simulink library "TorqueCommand"  (R2025a)
settings: Solver=VariableStepAuto  StartTime=0.0  StopTime=10.0  RelTol=1e-3
values from neighbouring files (symbols this model uses):
  RegenEnable : value not decoded    [TorqueCommand.sldd]
  TCEnable : value not decoded    [TorqueCommand.sldd]
undefined symbols (not defined in the file or in its folder): DiscIntNeverNeededParam, dt, raptor_xcp_function, TorqueKiLowerSat, TorqueKiUpperSat
libraries: Raptor_lib x56, Utilities x14, simulink x7, $bdroot x5
(part 2 of 2)

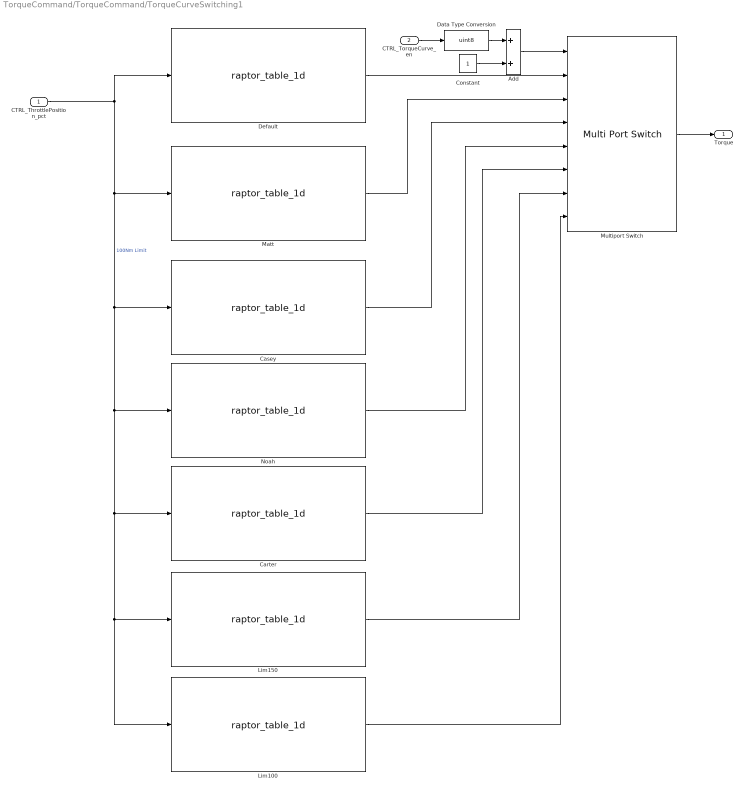
== system TorqueCommand/TorqueCommand/TorqueCurveSwitching1 ==
  CTRL_ThrottlePosition_pct : Inport
  CTRL_TorqueCurve_en : Inport  Port=2
  Add : Sum
  Carter : Raptor_lib/Table Lookup/raptor_table_1d  dataName='CTRL_ThrottleToTorqueCmdCarter_1D'  initValue=[0;1;3;6;11;18;25;34;45;57;70;85;101;118;137;158;179;202;227;230;230]  dataType=single  storage=Calibration  initValueX=[0;5;10;15;20;25;30;35;40;45;50;55;60;65;70;75;80;85;90;95;100]  dataTypeXY=single  storageXY=Calibration  calVisible=on  showTable=on  calGain=1.0  calOffset=0.0  calMax=Inf  calMin=-Inf  calFormat='-1'  calUnit='pct'  calHelp=''  showBreakpoint=on  dataNameX=[]  calGainX=1.0  calOffsetX=0.0  calMaxX=Inf  calMinX=-Inf  calFormatX='-1'  calUnitX='Nm'  calHelpX=''  calAccess=1  calFunction=raptor_xcp_function(gcb)  measureEnable=off  mName=['Data1D_Output']
      settings: SourceProductName=Raptor
  Casey : Raptor_lib/Table Lookup/raptor_table_1d  dataName='CTRL_ThrottleToTorqueCmdCasey_1D'  initValue=[0;3;6;9;12;15;25;35;45;55;65;75;85;95;105;115;135;155;175;195;200]  dataType=single  storage=Calibration  initValueX=[0;5;10;15;20;25;30;35;40;45;50;55;60;65;70;75;80;85;90;95;100]  dataTypeXY=single  storageXY=Calibration  calVisible=on  showTable=on  calGain=1.0  calOffset=0.0  calMax=Inf  calMin=-Inf  calFormat='-1'  calUnit='pct'  calHelp=''  showBreakpoint=on  dataNameX=[]  calGainX=1.0  calOffsetX=0.0  calMaxX=Inf  calMinX=-Inf  calFormatX='-1'  calUnitX='Nm'  calHelpX=''  calAccess=1  calFunction=raptor_xcp_function(gcb)  measureEnable=off  mName=['Data1D_Output']
      settings: SourceProductName=Raptor
  Constant : Constant
  Data Type Conversion : DataTypeConversion  OutDataTypeStr=uint8  SaturateOnIntegerOverflow=off  RndMeth=Floor
  Default : Raptor_lib/Table Lookup/raptor_table_1d  dataName='CTRL_ThrottleToTorqueCmdDef_1D'  initValue=[0;3;6;9;12;15;25;35;45;55;65;75;85;95;105;115;135;155;175;195;200]  dataType=single  storage=Calibration  initValueX=[0;5;10;15;20;25;30;35;40;45;50;55;60;65;70;75;80;85;90;95;100]  dataTypeXY=single  storageXY=Calibration  calVisible=on  showTable=on  calGain=1.0  calOffset=0.0  calMax=Inf  calMin=-Inf  calFormat='-1'  calUnit='pct'  calHelp=''  showBreakpoint=on  dataNameX=[]  calGainX=1.0  calOffsetX=0.0  calMaxX=Inf  calMinX=-Inf  calFormatX='-1'  calUnitX='Nm'  calHelpX=''  calAccess=1  calFunction=raptor_xcp_function(gcb)  measureEnable=off  mName=['Data1D_Output']
      settings: SourceProductName=Raptor
  Lim100 : Raptor_lib/Table Lookup/raptor_table_1d  dataName='CTRL_ThrottleToTorqueCmd100_1D'  initValue=[0;8;17;25;33;40;48;55;62;68;74;79;84;88;92;95;97;99;100;100;100]  dataType=single  storage=Calibration  initValueX=[0;5;10;15;20;25;30;35;40;45;50;55;60;65;70;75;80;85;90;95;100]  dataTypeXY=single  storageXY=Calibration  calVisible=on  showTable=on  calGain=1.0  calOffset=0.0  calMax=Inf  calMin=-Inf  calFormat='-1'  calUnit='pct'  calHelp=''  showBreakpoint=on  dataNameX=[]  calGainX=1.0  calOffsetX=0.0  calMaxX=Inf  calMinX=-Inf  calFormatX='-1'  calUnitX='Nm'  calHelpX=''  calAccess=1  calFunction=raptor_xcp_function(gcb)  measureEnable=off  mName=['Data1D_Output']
      settings: SourceProductName=Raptor
  Lim150 : Raptor_lib/Table Lookup/raptor_table_1d  dataName='CTRL_ThrottleToTorqueCmd150_1D'  initValue=[0;8;17;25;33;40;48;55;62;68;74;79;84;88;92;95;97;99;100;100;100]  dataType=single  storage=Calibration  initValueX=[0;5;10;15;20;25;30;35;40;45;50;55;60;65;70;75;80;85;90;95;100]  dataTypeXY=single  storageXY=Calibration  calVisible=on  showTable=on  calGain=1.0  calOffset=0.0  calMax=Inf  calMin=-Inf  calFormat='-1'  calUnit='pct'  calHelp=''  showBreakpoint=on  dataNameX=[]  calGainX=1.0  calOffsetX=0.0  calMaxX=Inf  calMinX=-Inf  calFormatX='-1'  calUnitX='Nm'  calHelpX=''  calAccess=1  calFunction=raptor_xcp_function(gcb)  measureEnable=off  mName=['Data1D_Output']
      settings: SourceProductName=Raptor
  Matt : Raptor_lib/Table Lookup/raptor_table_1d  dataName='CTRL_ThrottleToTorqueCmdMatt_1D'  initValue=[0;3;6;9;12;15;25;35;45;55;65;75;85;95;105;115;135;155;175;195;200]  dataType=single  storage=Calibration  initValueX=[0;5;10;15;20;25;30;35;40;45;50;55;60;65;70;75;80;85;90;95;100]  dataTypeXY=single  storageXY=Calibration  calVisible=on  showTable=on  calGain=1.0  calOffset=0.0  calMax=Inf  calMin=-Inf  calFormat='-1'  calUnit='pct'  calHelp=''  showBreakpoint=on  dataNameX=[]  calGainX=1.0  calOffsetX=0.0  calMaxX=Inf  calMinX=-Inf  calFormatX='-1'  calUnitX='Nm'  calHelpX=''  calAccess=1  calFunction=raptor_xcp_function(gcb)  measureEnable=off  mName=['Data1D_Output']
      settings: SourceProductName=Raptor
  Multiport Switch : MultiPortSwitch  Inputs=7  SaturateOnIntegerOverflow=off  InputSameDT=off
  Noah : Raptor_lib/Table Lookup/raptor_table_1d  dataName='CTRL_ThrottleToTorqueCmdNoah_1D'  initValue=[0;3;6;9;12;15;25;35;45;55;65;75;85;95;105;115;135;155;175;195;200]  dataType=single  storage=Calibration  initValueX=[0;5;10;15;20;25;30;35;40;45;50;55;60;65;70;75;80;85;90;95;100]  dataTypeXY=single  storageXY=Calibration  calVisible=on  showTable=on  calGain=1.0  calOffset=0.0  calMax=Inf  calMin=-Inf  calFormat='-1'  calUnit='pct'  calHelp=''  showBreakpoint=on  dataNameX=[]  calGainX=1.0  calOffsetX=0.0  calMaxX=Inf  calMinX=-Inf  calFormatX='-1'  calUnitX='Nm'  calHelpX=''  calAccess=1  calFunction=raptor_xcp_function(gcb)  measureEnable=off  mName=['Data1D_Output']
      settings: SourceProductName=Raptor
  Torque : Outport
  wires:
  Data Type Conversion/1 -> Add/1
  Constant/1 -> Add/2
  Add/1 -> Multiport Switch/1
  CTRL_TorqueCurve_en/1 -> Data Type Conversion/1
  Multiport Switch/1 -> Torque/1
  Lim100/1 -> Multiport Switch/8
  Lim150/1 -> Multiport Switch/7
  Carter/1 -> Multiport Switch/6
  Noah/1 -> Multiport Switch/5
  Casey/1 -> Multiport Switch/4
  Matt/1 -> Multiport Switch/3
  Default/1 -> Multiport Switch/2
  CTRL_ThrottlePosition_pct/1 -> Default/1, Matt/1, Casey/1, Noah/1, Carter/1, Lim100/1, Lim150/1  "100Nm Limit"

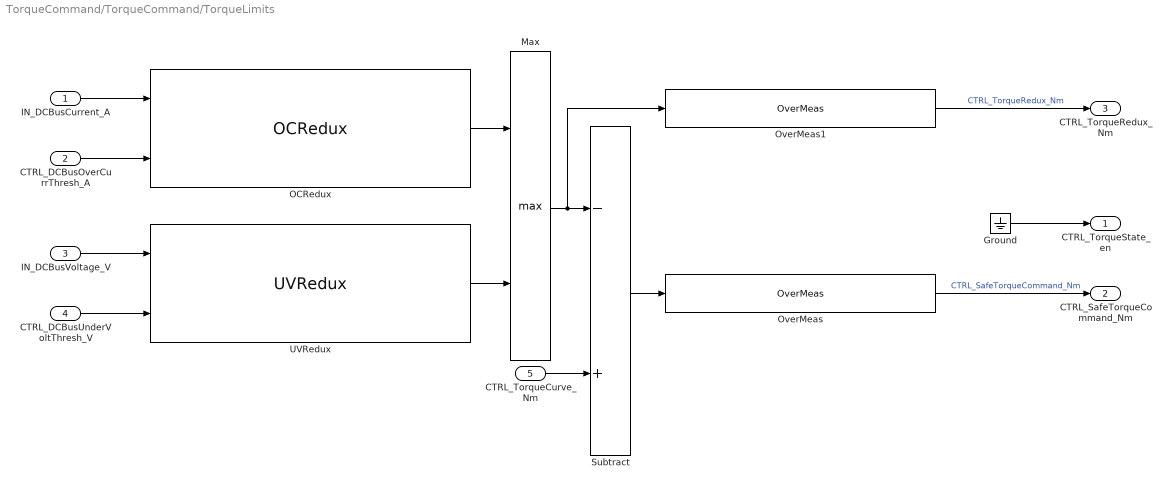
== system TorqueCommand/TorqueCommand/TorqueLimits ==
  IN_DCBusCurrent_A : Inport
  CTRL_DCBusOverCurrThresh_A : Inport  Port=2
  IN_DCBusVoltage_V : Inport  Port=3
  CTRL_DCBusUnderVoltThresh_V : Inport  Port=4
  CTRL_TorqueCurve_Nm : Inport  Port=5
  Ground : Ground
  Max : MinMax  Function=max  Inputs=2
  OCRedux : $bdroot/OCRedux  SystemSampleTime=-1  VariantActivationTime=update diagram  EmptyChoice=off  PassThrough=off  PassThroughVariantControl=(default)  EmptyChoiceVariantControl=(default)  AllowFlexibleInterface=on  Latency=0  AutoFrameSizeCalculation=off
  OverMeas : Utilities/OverMeas  sigName='CTRL_SafeTorqueCommand_Nm'  minimum=-inf  maximum=inf
  OverMeas1 : Utilities/OverMeas  sigName='CTRL_TorqueRedux_Nm'  minimum=-inf  maximum=inf
  Subtract : Sum  Inputs=-+
  UVRedux : $bdroot/UVRedux  SystemSampleTime=-1  VariantActivationTime=update diagram  EmptyChoice=off  PassThrough=off  PassThroughVariantControl=(default)  EmptyChoiceVariantControl=(default)  AllowFlexibleInterface=on  Latency=0  AutoFrameSizeCalculation=off
  CTRL_TorqueState_en : Outport
  CTRL_SafeTorqueCommand_Nm : Outport  Port=2
  CTRL_TorqueRedux_Nm : Outport  Port=3
  wires:
  OverMeas1/1 -> CTRL_TorqueRedux_Nm/1  "CTRL_TorqueRedux_Nm"
  Ground/1 -> CTRL_TorqueState_en/1
  CTRL_DCBusUnderVoltThresh_V/1 -> UVRedux/2
  IN_DCBusVoltage_V/1 -> UVRedux/1
  UVRedux/1 -> Max/2
  OverMeas/1 -> CTRL_SafeTorqueCommand_Nm/1  "CTRL_SafeTorqueCommand_Nm"
  Subtract/1 -> OverMeas/1
  CTRL_TorqueCurve_Nm/1 -> Subtract/2
  Max/1 -> Subtract/1, OverMeas1/1
  CTRL_DCBusOverCurrThresh_A/1 -> OCRedux/2
  IN_DCBusCurrent_A/1 -> OCRedux/1
  OCRedux/1 -> Max/1

== matlab function TorqueCommand/ShifterState/MATLAB Function ==
  data: IO_PwrUpSwitch_bool input; IO_PwrDownSwitch_bool input; stateNum output
function stateNum = fcn(IO_PwrUpSwitch_bool, IO_PwrDownSwitch_bool)
 
persistent state prevUp prevDown
 
if isempty(state)

    state = TorqueState.State5;

end

if isempty(prevUp)

    prevUp = false;

    prevDown = false;

end
 
upButton = logical(IO_PwrUpSwitch_bool);

downButton = logical(IO_PwrDownSwitch_bool);
 
upEdge = (upButton && ~prevUp);

downEdge = (downButton && ~prevDown);
 
if upEdge

    newValue = min(uint8(state) + 1, 5);

    state = TorqueState(newValue);

elseif downEdge

    newValue = max(uint8(state) - 1, 0);

    state = TorqueState(newValue);

end
 
stateNum = uint8(state);
 
prevUp = upButton;

prevDown = downButton;

== stateflow chart TorqueCommand/TorqueProfiles/Chart ==
  state VehicleStatic
    state Default
      entry:
      Profile = TorqueProfile.Player1;
      Curve = TorqueCurve.Default;
      TC = TCEnable.TCOff;
      Regen = RegenEnable.RegOff;
      Sensitivity = 5;
    state Testing2
      entry:
      Profile = TorqueProfile.Testing2;
      Curve = TorqueCurve.Lim100;
      TC = TCEnable.TCOn;
      Regen = RegenEnable.RegOn;
      Sensitivity = 5;
    state Driver1
      entry:
      Profile = TorqueProfile.Driver1;
      Curve = TorqueCurve.Matt;
      TC = TCEnable.TCOn;
      Regen = RegenEnable.RegOn;
      Sensitivity = 5;
    state Testing3
      entry:
      Profile = TorqueProfile.Testing3;
      Curve = TorqueCurve.Default;
      TC = TCEnable.TCOn;
      Regen = RegenEnable.RegOn;
      Sensitivity = 0;
    state Driver2
      entry:
      Profile = TorqueProfile.Driver2;
      Curve = TorqueCurve.Casey;
      TC = TCEnable.TCOn;
      Regen = RegenEnable.RegOn;
      Sensitivity = 5;
    state Testing4
      entry:
      Profile = TorqueProfile.Testing4;
      Curve = TorqueCurve.Default;
      TC = TCEnable.TCOn;
      Regen = RegenEnable.RegOn;
      Sensitivity = 1;
    state Driver3
      entry:
      Profile = TorqueProfile.Driver3;
      Curve = TorqueCurve.Noah;
      TC = TCEnable.TCOn;
      Regen = RegenEnable.RegOn;
      Sensitivity = 5;
    state Testing5
      entry:
      Profile = TorqueProfile.Testing5;
      Curve = TorqueCurve.Default;
      TC = TCEnable.TCOn;
      Regen = RegenEnable.RegOn;
      Sensitivity = 2;
    state Driver4
      entry:
      Profile = TorqueProfile.Driver4;
      Curve = TorqueCurve.Carter;
      TC = TCEnable.TCOn;
      Regen = RegenEnable.RegOn;
      Sensitivity = 5;
    state Testing6
      entry:
      Profile = TorqueProfile.Testing6;
      Curve = TorqueCurve.Default;
      TC = TCEnable.TCOn;
      Regen = RegenEnable.RegOn;
      Sensitivity = 3;
    state Testing1
      entry:
      Profile = TorqueProfile.Testing1;
      Curve = TorqueCurve.Lim150;
      TC = TCEnable.TCOn;
      Regen = RegenEnable.RegOn;
      Sensitivity = 5;
    (default) -> Default
    (junction 264) -> Default : [TCDial == 0]
    Testing2 -> (junction 276) : [TCDial ~= 6]
    (junction 47) -> (junction 264) [order 1]
    (junction 276) -> (junction 47)
    Default -> (junction 287) : [TCDial ~= 0]
    (junction 289) -> Testing2 : [TCDial == 6]
    (junction 287) -> (junction 47)
    (junction 47) -> (junction 289) [order 7]
    (junction 282) -> Driver1 : [TCDial == 1]
    Testing3 -> (junction 284) : [TCDial ~= 7]
    (junction 47) -> (junction 282) [order 2]
    (junction 284) -> (junction 47)
    Driver1 -> (junction 283) : [TCDial ~= 1]
    (junction 285) -> Testing3 : [TCDial == 7]
    (junction 283) -> (junction 47)
    (junction 47) -> (junction 285) [order 8]
    Testing4 -> (junction 269) : [TCDial ~= 8]
    (junction 273) -> Driver2 : [TCDial == 2]
    (junction 47) -> (junction 273) [order 3]
    (junction 269) -> (junction 47)
    (junction 274) -> (junction 47)
    (junction 47) -> (junction 267) [order 9]
    (junction 267) -> Testing4 : [TCDial == 8]
    (junction 47) -> (junction 271) [order 4]
    (junction 277) -> (junction 47)
    Driver2 -> (junction 274) : [TCDial ~= 2]
    (junction 272) -> (junction 47)
    (junction 47) -> (junction 278) [order 10]
    (junction 47) -> (junction 270) [order 5]
    (junction 280) -> (junction 47)
    (junction 268) -> (junction 47)
    (junction 47) -> (junction 279) [order 11]
    (junction 47) -> (junction 263) [order 6] : [TCDial == 5]
    (junction 281) -> (junction 47) : [TCDial ~= 5]
    (junction 271) -> Driver3 : [TCDial == 3]
    Testing5 -> (junction 277) : [TCDial ~= 9]
    Driver3 -> (junction 272) : [TCDial ~= 3]
    (junction 278) -> Testing5 : [TCDial == 9]
    (junction 270) -> Driver4 : [TCDial == 4]
    Testing6 -> (junction 280) : [TCDial ~= 10]
    Driver4 -> (junction 268) : [TCDial ~= 4]
    (junction 279) -> Testing6 : [TCDial == 10]
    (junction 263) -> Testing1
    Testing1 -> (junction 281)
  state ReadyToMove
    state NoTC
      entry:
      Sensitivity = 1;
    state Sens6
      entry:
      Sensitivity = 6;
    state Sens7
      entry:
      Sensitivity = 7;
    state Sens1
      entry:
      Sensitivity = 2;
    state Sens2
      entry:
      Sensitivity = 2;
    state Sens8
      entry:
      Sensitivity = 8;
    state Sens3
      entry:
      Sensitivity = 3;
    state Sens9
      entry:
      Sensitivity = 9;
    state Sens4
      entry:
      Sensitivity = 4;
    state Sens10
      entry:
      Sensitivity = 10;
    state Sens5
      entry:
      Sensitivity = 5;
    (default) -> NoTC
    (junction 395) -> NoTC : [TCDial == 0]
    Sens6 -> (junction 391) : [TCDial ~= 6]
    (junction 403) -> (junction 395) [order 1]
    (junction 391) -> (junction 403)
    NoTC -> (junction 396) : [TCDial ~= 0]
    (junction 397) -> Sens6 : [TCDial == 6]
    (junction 396) -> (junction 403)
    (junction 403) -> (junction 397) [order 7]
    (junction 390) -> Sens1 : [TCDial == 1]
    Sens7 -> (junction 392) : [TCDial ~= 7]
    (junction 403) -> (junction 390) [order 2]
    (junction 392) -> (junction 403)
    Sens1 -> (junction 394) : [TCDial ~= 1]
    (junction 393) -> Sens7 : [TCDial == 7]
    (junction 394) -> (junction 403)
    (junction 403) -> (junction 393) [order 8]
    Sens8 -> (junction 398) : [TCDial ~= 8]
    (junction 402) -> Sens2 : [TCDial == 2]
    (junction 403) -> (junction 402) [order 3]
    (junction 398) -> (junction 403)
    (junction 399) -> (junction 403)
    (junction 403) -> (junction 407) [order 9]
    (junction 407) -> Sens8 : [TCDial == 8]
    (junction 403) -> (junction 400) [order 4]
    (junction 401) -> (junction 403)
    Sens2 -> (junction 399) : [TCDial ~= 2]
    (junction 404) -> (junction 403)
    (junction 403) -> (junction 405) [order 10]
    (junction 403) -> (junction 406) [order 5]
    (junction 408) -> (junction 403)
    (junction 409) -> (junction 403)
    (junction 403) -> (junction 413) [order 11]
    (junction 403) -> (junction 410) [order 6]
    (junction 411) -> (junction 403)
    (junction 400) -> Sens3 : [TCDial == 3]
    Sens9 -> (junction 401) : [TCDial ~= 9]
    Sens3 -> (junction 404) : [TCDial ~= 3]
    (junction 405) -> Sens9 : [TCDial == 9]
    (junction 406) -> Sens4 : [TCDial == 4]
    Sens10 -> (junction 408) : [TCDial ~= 10]
    Sens4 -> (junction 409) : [TCDial ~= 4]
    (junction 413) -> Sens10 : [TCDial == 10]
    (junction 410) -> Sens5 : [TCDial == 5]
    Sens5 -> (junction 411) : [TCDial ~= 5]
  (default) -> VehicleStatic
  VehicleStatic -> ReadyToMove : [[State == VehicleState.ReadyToMove]]
  ReadyToMove -> VehicleStatic : [State ~= VehicleState.ReadyToMove]
  data: Profile output; Curve output; Sensitivity output; TCDial input; State input; Regen output; TC output

== stateflow chart TorqueCommand/BrakeRegen/Chart ==
  state RegenOff
    en:
    RegenMode = 0;
  state RegenOn
    state RegenMode1
      en:
      RegenMode = 1;
      RegenCoefficient = 1;
    state RegenMode2
      en:
      RegenMode = 2;
      RegenCoefficient = 1.5;
    state RegenMode4
      en:
      RegenMode = 4;
      RegenCoefficient = 2.5;
    state RegenMode3
      en:
      RegenMode = 3;
      RegenCoefficient = 2;
    state RegenMode5
      en:
      RegenMode = 5;
      RegenCoefficient = 3;
    state RegenMode6
      en:
      RegenMode = 6;
      RegenCoefficient = 3.5;
    state RegenMode7
      en:
      RegenMode = 7;
      RegenCoefficient = CTRL_RegenCoefficient_int;
    (default) -> RegenMode1
    RegenMode2 -> RegenMode1 [order 1] : [CTRL_DebPwrDown_int == 1]
    RegenMode1 -> RegenMode2 : [CTRL_DebPwrUp_int == 1]
    RegenMode3 -> RegenMode2 [order 1] : [CTRL_DebPwrDown_int == 1]
    RegenMode2 -> RegenMode3 [order 2] : [CTRL_DebPwrUp_int == 1]
    RegenMode3 -> RegenMode4 [order 2] : [CTRL_DebPwrUp_int == 1]
    RegenMode4 -> RegenMode3 [order 1] : [CTRL_DebPwrDown_int == 1]
    RegenMode5 -> RegenMode4 [order 1] : [CTRL_DebPwrDown_int == 1]
    RegenMode4 -> RegenMode5 [order 2] : [CTRL_DebPwrUp_int == 1]
    RegenMode5 -> RegenMode6 [order 2] : [CTRL_DebPwrUp_int == 1]
    RegenMode6 -> RegenMode5 [order 1] : [CTRL_DebPwrDown_int == 1]
    RegenMode7 -> RegenMode6 : [CTRL_DebPwrDown_int == 1]
    RegenMode6 -> RegenMode7 [order 2] : [CTRL_DebPwrUp_int == 1]
  (default) -> RegenOff
  RegenOn -> RegenOff : [Regen == RegenEnable.RegOff && ...
      |  IN_DCBusVolt_V > 370 && ...
      | CTRL_ThrottlePosition_pct > 5 && ...
      | IN_MotorSpeed_rpm < 700]
  RegenOff -> RegenOn : [Regen == RegenEnable.RegOn && ...
      | IN_DCBusVolt_V <= 370 && ...
      | CTRL_ThrottlePosition_pct <= 5 && ...
      | IN_MotorSpeed_rpm >= 700]
  data: Regen input; IN_DCBusVolt_V input; CTRL_ThrottlePosition_pct input; CTRL_DebPwrUp_int input; CTRL_DebPwrDown_int input; RegenMode output; RegenCoefficient output; CTRL_RegenCoefficient_int input; IN_MotorSpeed_rpm input

== stateflow chart TorqueCommand/TorqueCeiling ==
  state Default
    en:
    State = TorqueCeiling.NA;
    Torque = 230;
  state UnderVoltage
    en:
    State = TorqueCeiling.UnderVoltage;
    state UnderVoltInit
      en:
      Torque = 100;
    state UnderVolt3
      en:
      Torque = 50;
    state UnderVolt2
      en:
      Torque = 50;
    (default) -> UnderVoltInit
    UnderVoltInit -> UnderVolt3 : [DCBusVolts >= UnderVoltageThreshold]
    UnderVolt3 -> UnderVolt2 : [DCBusVolts >= UnderVoltageThreshold]
  state OverCurrent1
    en:
    State = TorqueCeiling.OverCurr;
    state OverCurrInit
      en:
      Torque = 100;
    state OverCurr2
      en:
      Torque = 70;
    state OverCurr3
      en:
      Torque = 50;
    (default) -> OverCurrInit
    OverCurrInit -> OverCurr2 : [DCBusCurrent >= OverCurrentThreshold]
    OverCurr2 -> OverCurr3 : [DCBusCurrent >= OverCurrentThreshold]
  (default) -> Default
  Default -> (junction 31) [order 2] : [DCBusVolts >= UnderVoltageThreshold]
  Default -> (junction 18) [order 1] : [DCBusCurrent >= OverCurrentThreshold]
  (junction 31) -> UnderVoltage
  (junction 18) -> OverCurrent1
  (junction 34) -> Default
  UnderVoltage -> (junction 34) : [ThrottlePosition <= 50]
  OverCurrent1 -> (junction 34) : [ThrottlePosition <= 50]
  data: DCBusVolts input; DCBusCurrent input; ThrottlePosition input; UnderVoltageThreshold input; OverCurrentThreshold input; State output; Torque output

== matlab function TorqueCommand/BrakeRegen/MATLAB Function ==
  data: IO_PwrUpSwitch_bool input; CTRL_DebPwrUp_int output; IO_PwrDownSwitch_bool input; dt input; CTRL_DebPwrDown_int output
function [CTRL_DebPwrUp_int, CTRL_DebPwrDown_int] = debouncePowerButtons(IO_PwrUpSwitch_bool, IO_PwrDownSwitch_bool, dt)
% Debounce two power buttons
%
% Inputs:
%   IO_PwrUpSwitch_bool   - raw Power Up button input
%   IO_PwrDownSwitch_bool - raw Power Down button input
%   dt                    - sample time in seconds
%
% Outputs:
%   CTRL_DebPwrUp_int     - debounced Power Up button
%   CTRL_DebPwrDown_int   - debounced Power Down button

    persistent upOut upLastRaw upCount
    persistent downOut downLastRaw downCount

    debounceTime = 0.03;   % 30 ms debounce
    nDebounce = max(1, ceil(debounceTime / dt));

    if isempty(upOut)
        upOut = logical(IO_PwrUpSwitch_bool);
        upLastRaw = logical(IO_PwrUpSwitch_bool);
        upCount = 0;

        downOut = logical(IO_PwrDownSwitch_bool);
        downLastRaw = logical(IO_PwrDownSwitch_bool);
        downCount = 0;
    end

    % -------- Power Up debounce --------
    rawUp = logical(IO_PwrUpSwitch_bool);

    if rawUp ~= upLastRaw
        upLastRaw = rawUp;
        upCount = 1;
    else
        upCount = upCount + 1;
    end

    if rawUp ~= upOut && upCount >= nDebounce
        upOut = rawUp;
    end

    % -------- Power Down debounce --------
    rawDown = logical(IO_PwrDownSwitch_bool);

    if rawDown ~= downLastRaw
        downLastRaw = rawDown;
        downCount = 1;
    else
        downCount = downCount + 1;
    end

    if rawDown ~= downOut && downCount >= nDebounce
        downOut = rawDown;
    end

    CTRL_DebPwrUp_int = upOut;
    CTRL_DebPwrDown_int = downOut;
end
